simulink model "FuzzyController"  (R2024a)
settings: Solver=VariableStepAuto  StartTime=0.0  StopTime=10.0  RelTol=1e-3
libraries: fuzblock x1
settings Model: Creator=max11mus  LastModifiedBy=max11mus

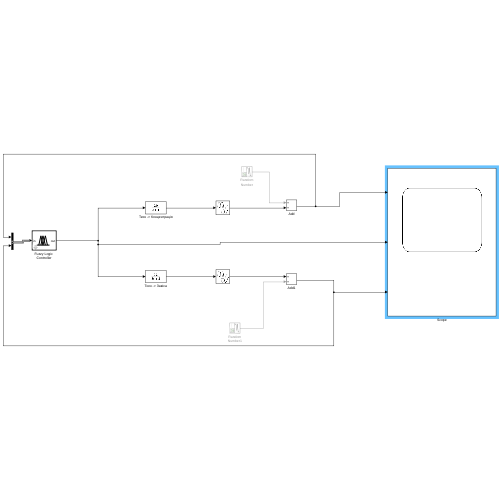
[thumbnail: Simulink's stored preview of the top-level diagram]
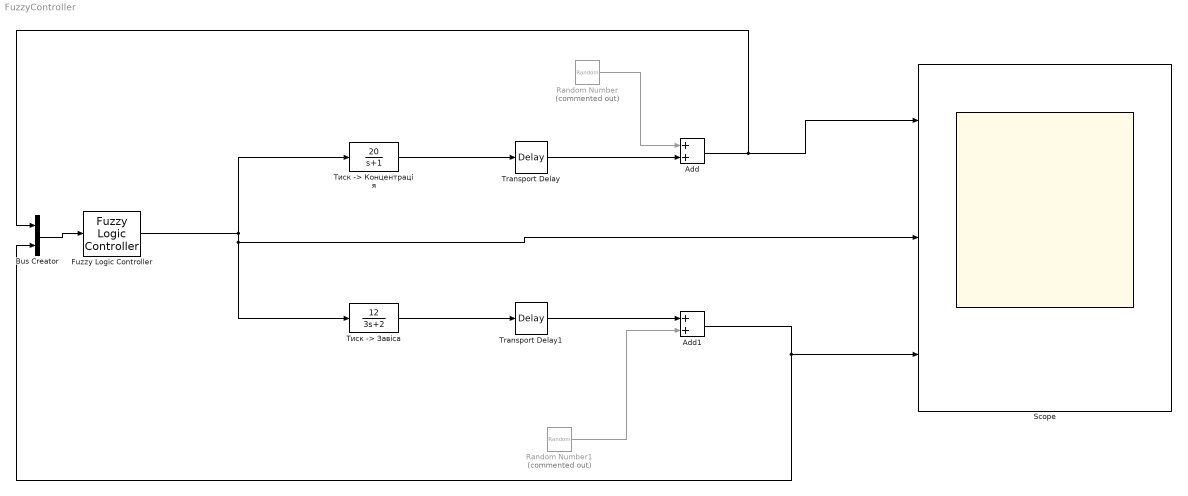
== system FuzzyController ==
  Add : Sum
  Add1 : Sum
  Bus Creator : BusCreator  Inputs=2
  Fuzzy Logic Controller : fuzblock/Fuzzy Logic  Controller  FIS='Mamdani.fis'  OutputSampleNumber=101  DataType=double  FuzzifiedInputs=off  RuleFiringStrengths=off  RuleOutputs=off  AggregatedOutputs=off  SimulateUsing=Interpreted execution  OutOfRangeInputValueMessage=warning  NoRuleFiredMessage=warning  EmptyOutputFuzzySetMessage=warning
  Random Number : RandomNumber  Commented=on  SampleTime=0.1
  Random Number1 : RandomNumber  Commented=on  SampleTime=0.1
  Scope : Scope  NumInputPorts=3
  Transport Delay : TransportDelay
  Transport Delay1 : TransportDelay
  "Тиск -> Завіса" : TransferFcn  Numerator=[12]  Denominator=[3 2]
  "Тиск -> Концентрація" : TransferFcn  Numerator=[20]  Denominator=[1 1]
  wires:
  Fuzzy Logic Controller/1 -> Scope/2, "Тиск -> Завіса"/1, "Тиск -> Концентрація"/1
  "Тиск -> Концентрація"/1 -> Transport Delay/1
  Transport Delay/1 -> Add/2
  Random Number/1 -> Add/1
  "Тиск -> Завіса"/1 -> Transport Delay1/1
  Transport Delay1/1 -> Add1/1
  Random Number1/1 -> Add1/2
  Bus Creator/1 -> Fuzzy Logic Controller/1
  Add1/1 -> Bus Creator/2, Scope/3
  Add/1 -> Scope/1, Bus Creator/1
